simulink model "exnb4137986_Q8"  (R2024b)
settings: Solver=FixedStepAuto  StartTime=0.0  StopTime=300  FixedStep=0.001  RelTol=1e-3
values from neighbouring files (symbols this model uses):
  K = place(A, B, lambda_cl)    [exnb4137986_Q6_par.m]    (also in exnb4137986_Q8_par.m; exnb4137986_Q9_par.m)
  lambda_cl = [-10, -11]    [exnb4137986_Q6_par.m]    (also in exnb4137986_Q8_par.m; exnb4137986_Q9_par.m)
  m_star_1 = double(subs(m, x2, omega_star_1))    [exnb4137986_Q4_par.m]    (also in exnb4137986_Q6_par.m; exnb4137986_Q8_par.m; exnb4137986_Q9_par.m)
  m_star_2 = double(subs(m, x2, omega_star_2))    [exnb4137986_Q4_par.m]    (also in exnb4137986_Q6_par.m; exnb4137986_Q8_par.m; exnb4137986_Q9_par.m)
  omega_star_1 = 200    [exnb4137986_Q4_par.m]    (also in exnb4137986_Q6_par.m; exnb4137986_Q8_par.m; exnb4137986_Q9_par.m)
  omega_star_2 = 300    [exnb4137986_Q4_par.m]    (also in exnb4137986_Q6_par.m; exnb4137986_Q8_par.m; exnb4137986_Q9_par.m)
  r = 300    [exnb4137986_Q8_par.m]    (also in exnb4137986_Q9_par.m)
  u_star_1 = double(subs(u, x2, omega_star_1))    [exnb4137986_Q4_par.m]    (also in exnb4137986_Q6_par.m; exnb4137986_Q8_par.m; exnb4137986_Q9_par.m)
  values = [1, 10, 0.1, 40]    [exnb4137986_Q4_par.m]    (also in exnb4137986_Q6_par.m; exnb4137986_Q8_par.m; exnb4137986_Q9_par.m)
settings Model: Creator=therkelsen  LastModifiedBy=therkelsen

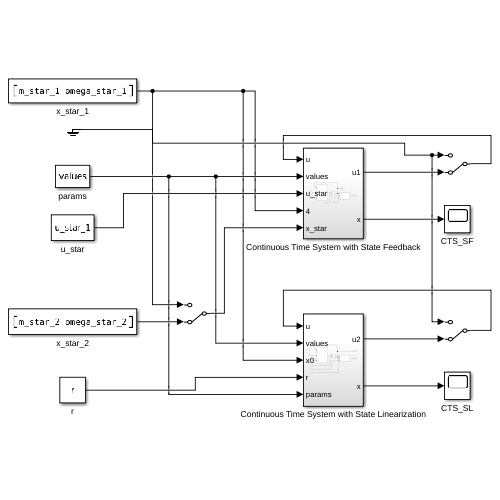
[thumbnail: Simulink's stored preview of the top-level diagram]
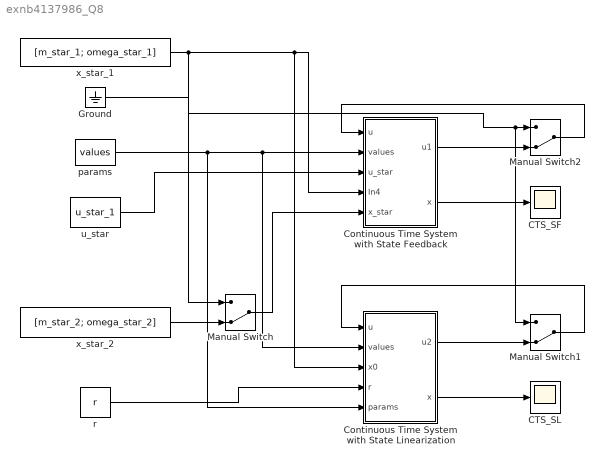
== system exnb4137986_Q8 ==
  CTS_SF : Scope
  CTS_SL : Scope
  Continuous Time System with State Feedback : Subsystem
  Continuous Time System with State Linearization : Subsystem
  Ground : Ground
  Manual Switch : ManualSwitch  CurrentSetting=0
  Manual Switch1 : ManualSwitch  CurrentSetting=0
  Manual Switch2 : ManualSwitch  CurrentSetting=0
  params : Constant  Value=values
  r : Constant  Value=r
  u_star : Constant  Value=u_star_1
  x_star_1 : Constant  Value=[m_star_1; omega_star_1]
  x_star_2 : Constant  Value=[m_star_2; omega_star_2]
  wires:
  x_star_2/1 -> Manual Switch/2
  Continuous Time System with State Feedback/2(x) -> CTS_SF/1
  Manual Switch2/1 -> Continuous Time System with State Feedback/1(u)
  params/1 -> Continuous Time System with State Linearization/5(params), Continuous Time System with State Linearization/2(values), Continuous Time System with State Feedback/2(values)
  u_star/1 -> Continuous Time System with State Feedback/3(u_star)
  Manual Switch/1 -> Continuous Time System with State Feedback/5(x_star)
  Ground/1 -> Manual Switch1/1, Manual Switch2/1
  Continuous Time System with State Linearization/2(x) -> CTS_SL/1
  Continuous Time System with State Feedback/1(u1) -> Manual Switch2/2
  x_star_1/1 -> Continuous Time System with State Linearization/3(x0), Continuous Time System with State Feedback/4(In4), Manual Switch/1
  Continuous Time System with State Linearization/1(u2) -> Manual Switch1/2
  Manual Switch1/1 -> Continuous Time System with State Linearization/1(u)
  r/1 -> Continuous Time System with State Linearization/4(r)

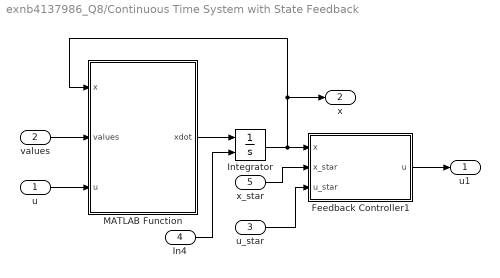
== system exnb4137986_Q8/Continuous Time System with State Feedback ==
  u : Inport
  values : Inport  Port=2
  u_star : Inport  Port=3
  In4 : Inport  Port=4
  x_star : Inport  Port=5
  Feedback Controller1 : Subsystem
  Integrator : Integrator  InitialConditionSource=external
  MATLAB Function : MATLAB Function  TreatAsAtomicUnit=on
  u1 : Outport
  x : Outport  Port=2
  wires:
  Feedback Controller1/1(u) -> u1/1
  Integrator/1 -> x/1, MATLAB Function/1(x), Feedback Controller1/1(x)
  In4/1 -> Integrator/2
  u_star/1 -> Feedback Controller1/3(u_star)
  x_star/1 -> Feedback Controller1/2(x_star)
  MATLAB Function/1(xdot) -> Integrator/1
  u/1 -> MATLAB Function/3(u)
  values/1 -> MATLAB Function/2(values)

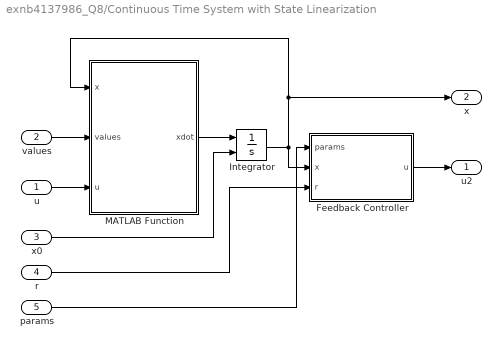
== system exnb4137986_Q8/Continuous Time System with State Linearization ==
  u : Inport
  values : Inport  Port=2
  x0 : Inport  Port=3
  r : Inport  Port=4
  params : Inport  Port=5
  Feedback Controller : Subsystem
  Integrator : Integrator  InitialConditionSource=external
  MATLAB Function : MATLAB Function  TreatAsAtomicUnit=on
  u2 : Outport
  x : Outport  Port=2
  wires:
  Feedback Controller/1(u) -> u2/1
  Integrator/1 -> Feedback Controller/2(x), x/1, MATLAB Function/1(x)
  x0/1 -> Integrator/2
  MATLAB Function/1(xdot) -> Integrator/1
  u/1 -> MATLAB Function/3(u)
  values/1 -> MATLAB Function/2(values)
  r/1 -> Feedback Controller/3(r)
  params/1 -> Feedback Controller/1(params)

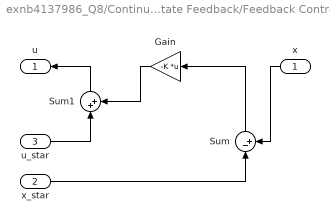
== system exnb4137986_Q8/Continuous Time System with State Feedback/Feedback Controller1 ==
  x : Inport
  x_star : Inport  Port=2
  u_star : Inport  Port=3
  Gain : Gain  Gain=-K  Multiplication=Matrix(K*u)
  Sum : Sum  Inputs=|-+
  Sum1 : Sum  Inputs=|++
  u : Outport
  wires:
  x/1 -> Sum/2
  Gain/1 -> Sum1/2
  Sum/1 -> Gain/1
  x_star/1 -> Sum/1
  u_star/1 -> Sum1/1
  Sum1/1 -> u/1

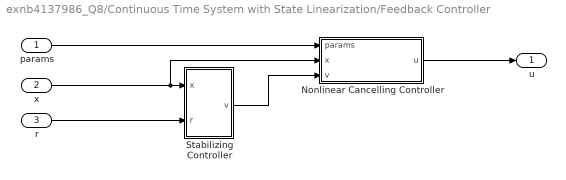
== system exnb4137986_Q8/Continuous Time System with State Linearization/Feedback Controller ==
  params : Inport
  x : Inport  Port=2
  r : Inport  Port=3
  Nonlinear Cancelling Controller : Subsystem
  Stabilizing Controller : Subsystem
  u : Outport
  wires:
  x/1 -> Nonlinear Cancelling Controller/2(x), Stabilizing Controller/1(x)
  r/1 -> Stabilizing Controller/2(r)
  Stabilizing Controller/1(v) -> Nonlinear Cancelling Controller/3(v)
  Nonlinear Cancelling Controller/1(u) -> u/1
  params/1 -> Nonlinear Cancelling Controller/1(params)

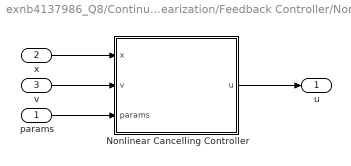
== system exnb4137986_Q8/Continuous Time System with State Linearization/Feedback Controller/Nonlinear Cancelling Controller ==
  params : Inport
  x : Inport  Port=2
  v : Inport  Port=3
  Nonlinear Cancelling Controller : MATLAB Function  TreatAsAtomicUnit=on
  u : Outport
  wires:
  v/1 -> Nonlinear Cancelling Controller/2(v)
  x/1 -> Nonlinear Cancelling Controller/1(x)
  params/1 -> Nonlinear Cancelling Controller/3(params)
  Nonlinear Cancelling Controller/1(u) -> u/1

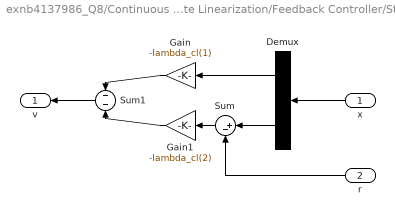
== system exnb4137986_Q8/Continuous Time System with State Linearization/Feedback Controller/Stabilizing Controller ==
  x : Inport
  r : Inport  Port=2
  Demux : Demux  Outputs=2
  Gain : Gain  Gain=-lambda_cl(1)
  Gain1 : Gain  Gain=-lambda_cl(2)
  Sum : Sum  Inputs=|+-
  Sum1 : Sum  Inputs=-|-
  v : Outport
  wires:
  Demux/2 -> Sum/1
  Gain/1 -> Sum1/1
  Sum/1 -> Gain1/1
  Gain1/1 -> Sum1/2
  r/1 -> Sum/2
  Demux/1 -> Gain/1
  x/1 -> Demux/1
  Sum1/1 -> v/1

== matlab function exnb4137986_Q8/Continuous Time System with State Feedback/MATLAB Function ==
  data: x input; values input; u input; xdot output
function xdot = fcn(x, values, u)

q1 = values(1);
q2 = values(2);
q3 = values(3);
J = values(4);

xdot = [-q1*x(2)*x(1) + u;
         q2/J*x(1) - q3/J*x(2)];

== matlab function exnb4137986_Q8/Continuous Time System with State Linearization/Feedback Controller/Nonlinear Cancelling Controller/Nonlinear Cancelling Controller ==
  data: x input; v input; u output; params input
function u = c_lin(x, v, params)

q1 = params(1);

u = q1*x(1)*x(2) + v;

== matlab function exnb4137986_Q8/Continuous Time System with State Linearization/MATLAB Function ==
  data: x input; values input; u input; xdot output
function xdot = fcn(x, values, u)

q1 = values(1);
q2 = values(2);
q3 = values(3);
J = values(4);

xdot = [-q1*x(2)*x(1) + u;
         q2/J*x(1) - q3/J*x(2)];
